simulink model "QuarterCar_2DOF"  (R2025b)
settings: Solver=VariableStepAuto  StartTime=0.0  StopTime=10.0  RelTol=1e-3
undefined symbols (not defined in the file): cs, ks, kt, m1, m2
settings Model: Creator=Aditya  LastModifiedBy=Aditya

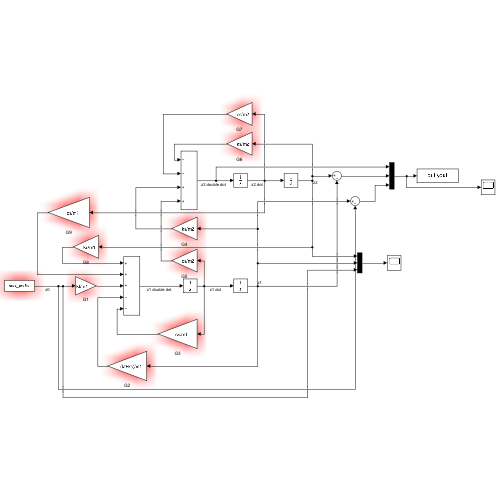
[thumbnail: Simulink's stored preview of the top-level diagram]
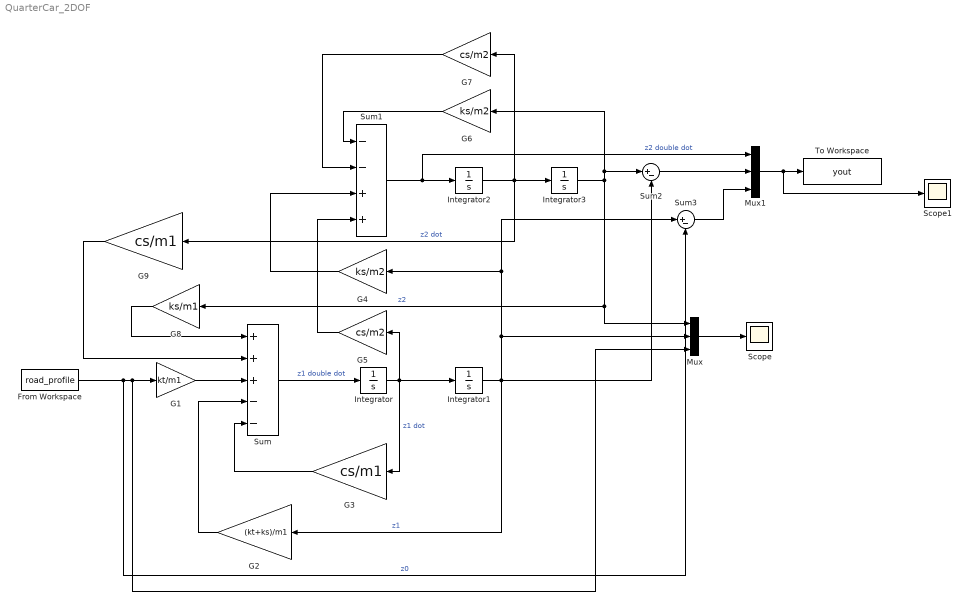
== system QuarterCar_2DOF ==
  From Workspace : FromWorkspace  VariableName=road_profile
  G1 : Gain  Gain=kt/m1
  G2 : Gain  Gain=(kt+ks)/m1
  G3 : Gain  Gain=cs/m1
  G4 : Gain  Gain=ks/m2
  G5 : Gain  Gain=cs/m2
  G6 : Gain  Gain=ks/m2
  G7 : Gain  Gain=cs/m2
  G8 : Gain  Gain=ks/m1
  G9 : Gain  Gain=cs/m1
  Integrator{,1..3} (4 alike) : Integrator
  Mux : Mux  Inputs=3
  Mux1 : Mux  Inputs=3
  Scope : Scope
      settings: ActiveDisplayYMinimum=-0.010688747849623113  ActiveDisplayYMaximum=0.096198730646608041
  Scope1 : Scope
      settings: ActiveDisplayYMinimum=-4.1926476137021336  ActiveDisplayYMaximum=3.1933082730436495
  Sum : Sum  Inputs=+++--
  Sum1 : Sum  Inputs=--++
  Sum2 : Sum  Inputs=|+-
  Sum3 : Sum  Inputs=|+-
  To Workspace : ToWorkspace  VariableName=yout  SaveFormat=Structure With Time  SampleTime=-1
  wires:
  From Workspace/1 -> Sum3/2, Mux/3, G1/1  "z0"
  G1/1 -> Sum/3
  Sum/1 -> Integrator/1  "z1 double dot"
  Integrator/1 -> G5/1, G3/1, Integrator1/1  "z1 dot"
  Integrator1/1 -> Sum3/1, G4/1, Mux/2, Sum2/2, G2/1  "z1"
  G2/1 -> Sum/4
  G3/1 -> Sum/5
  G4/1 -> Sum1/3
  G5/1 -> Sum1/4
  Sum1/1 -> Mux1/1, Integrator2/1  "z2 double dot"
  Integrator2/1 -> G9/1, G7/1, Integrator3/1  "z2 dot"
  Integrator3/1 -> Sum2/1, G6/1, Mux/1, G8/1  "z2"
  G6/1 -> Sum1/1
  G7/1 -> Sum1/2
  G8/1 -> Sum/1
  G9/1 -> Sum/2
  Mux/1 -> Scope/1
  Sum2/1 -> Mux1/2
  Sum3/1 -> Mux1/3
  Mux1/1 -> Scope1/1, To Workspace/1
